simulink model "Dynamics_M5"  (R2022b)
settings: Solver=ode4  StartTime=0.0  StopTime=300  FixedStep=0.01  RelTol=1e-3
settings Model: Creator=Abdullah Abdelaziz  LastModifiedBy=Abdullah Abdelaziz

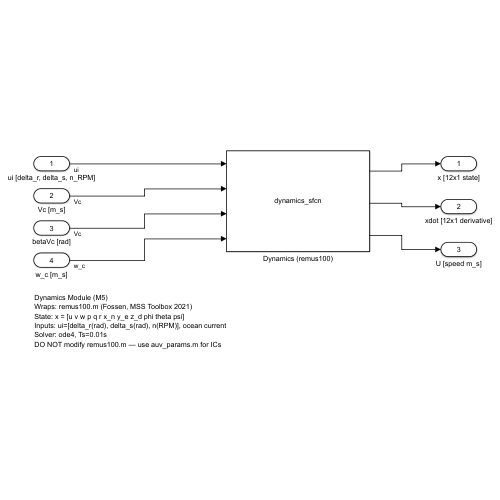
[thumbnail: Simulink's stored preview of the top-level diagram]
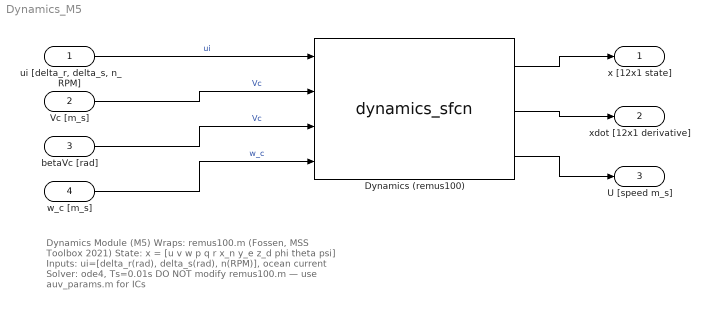
== system Dynamics_M5 ==
  note: Dynamics Module (M5)
      | Wraps: remus100.m (Fossen, MSS Toolbox 2021)
      | State: x = [u v w p q r x_n y_e z_d phi theta psi]
      | Inputs: ui=[delta_r(rad), delta_s(rad), n(RPM)], ocean current
      | Solver: ode4, Ts=0.01s
      | DO NOT modify remus100.m — use auv_params.m for ICs
  "ui [delta_r, delta_s, n_RPM]" : Inport  OutDataTypeStr=double  PortDimensions=3
  Vc [m_s] : Inport  Port=2  OutDataTypeStr=double  PortDimensions=1
  betaVc [rad] : Inport  Port=3  OutDataTypeStr=double  PortDimensions=1
  w_c [m_s] : Inport  Port=4  OutDataTypeStr=double  PortDimensions=1
  Dynamics (remus100) : M-S-Function  FunctionName=dynamics_sfcn
  x [12x1 state] : Outport  PortDimensions=12
  xdot [12x1 derivative] : Outport  Port=2  PortDimensions=12
  U [speed m_s] : Outport  Port=3  PortDimensions=1
  wires:
  "ui [delta_r, delta_s, n_RPM]"/1 -> Dynamics (remus100)/1  "ui"
  Vc [m_s]/1 -> Dynamics (remus100)/2  "Vc"
  betaVc [rad]/1 -> Dynamics (remus100)/3  "Vc"
  w_c [m_s]/1 -> Dynamics (remus100)/4  "w_c"
  Dynamics (remus100)/1 -> x [12x1 state]/1
  Dynamics (remus100)/2 -> xdot [12x1 derivative]/1
  Dynamics (remus100)/3 -> U [speed m_s]/1
